simulink model "limit_detection_test"  (R2013a)
settings: Solver=ode3  StartTime=0  StopTime=10000  FixedStep=1  RelTol=1e-3
libraries: simulink x1
settings Model: Creator=sfrank1  LastModifiedBy=sfrank1

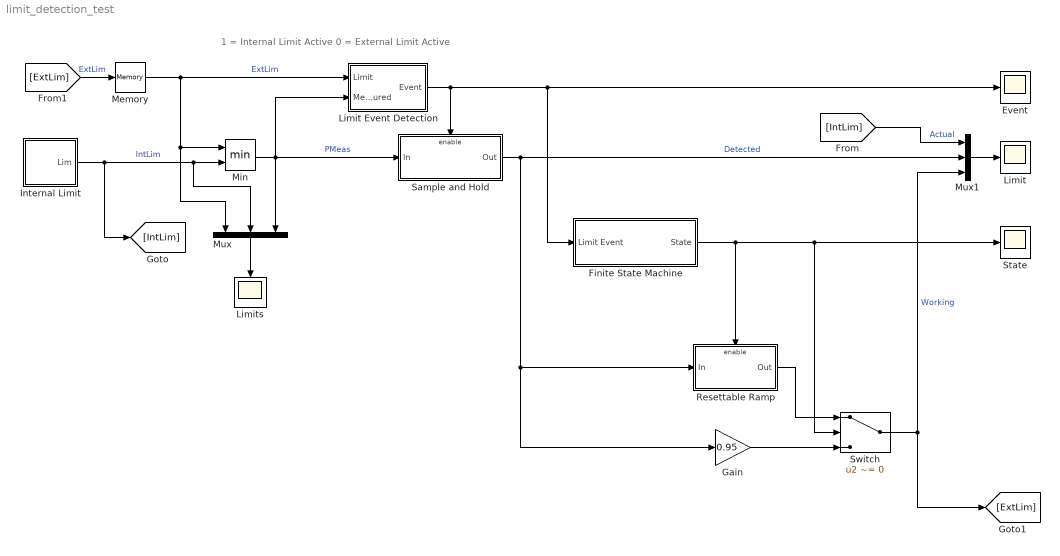
== system limit_detection_test ==
  note: 1 = Internal Limit Active
      | 0 = External Limit Active
  Event : Scope
      settings: TimeRange=10000  YMin=0  YMax=1
  Finite State Machine : Subsystem  TreatAsAtomicUnit=on
      settings: RTWFcnNameOpts=Use subsystem name  RTWFileNameOpts=Use function name
  Gain : Gain  Gain=0.95
  Internal Limit : Subsystem  TreatAsAtomicUnit=on
      settings: RTWFcnNameOpts=Use subsystem name  RTWFileNameOpts=Use function name
  Limit : Scope
      settings: ShowLegends=on  TimeRange=10000  YMin=0  YMax=2000  SaveName=ScopeData2
  Limit Event Detection : Subsystem  TreatAsAtomicUnit=on
      settings: RTWFcnNameOpts=Use subsystem name  RTWFileNameOpts=Use function name
  Limits : Scope
      settings: ShowLegends=on  TimeRange=10000  YMin=0  YMax=2000
  Memory : Memory
  Min : MinMax  Inputs=2
  Mux : Mux  Inputs=3
  Mux1 : Mux  Inputs=3
  Resettable Ramp : Subsystem  TreatAsAtomicUnit=on
  Sample and Hold : Subsystem  TreatAsAtomicUnit=on
  State : Scope
      settings: TimeRange=10000  YMin=0  YMax=1  SaveName=ScopeData4
  Switch : Switch  Criteria=u2 ~= 0
  wires:
  [ExtLim] -> Memory/1  "ExtLim"
  Min/1 -> Mux/3, Sample and Hold/1(In), Limit Event Detection/2(Measured)  "PMeas"
  Limit Event Detection/1(Event) -> Finite State Machine/1(Limit Event), Event/1, Sample and Hold/Enable
  Internal Limit/1(Lim) -> [IntLim], Mux/2, Min/2  "IntLim"
  Mux/1 -> Limits/1
  Finite State Machine/1(State) -> Switch/2, State/1, Resettable Ramp/Enable
  Resettable Ramp/1(Out) -> Switch/1
  Switch/1 -> [ExtLim], Mux1/3  "Working"
  Mux1/1 -> Limit/1
  [IntLim] -> Mux1/1  "Actual"
  Sample and Hold/1(Out) -> Mux1/2, Resettable Ramp/1(In), Gain/1  "Detected"
  Memory/1 -> Limit Event Detection/1(Limit), Mux/1, Min/1  "ExtLim"
  Gain/1 -> Switch/3

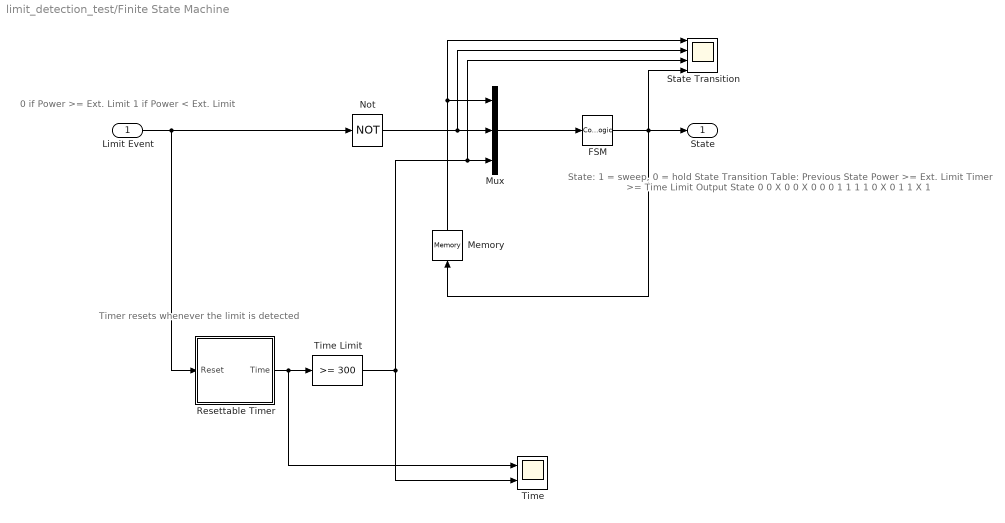
== system limit_detection_test/Finite State Machine ==
  note: Timer resets whenever the limit is detected
  note: 0 if Power >= Ext. Limit
      | 1 if Power < Ext. Limit
  note: State: 1 = sweep, 0 = hold
      |
      | State Transition Table:
      |
      | Previous State	Power >= Ext. Limit	Timer  >= Time Limit		Output State
      | 0				0					X						0
      | 0				X					0						0
      | 0				1					1						1
      | 1				0					X						0
      | 1				1					X						1
  Limit Event : Inport
  FSM : CombinatorialLogic  TruthTable=[0; 0; 0; 1; 0; 0; 1; 1]
  Memory : Memory  X0=1
  Mux : Mux  Inputs=3
  Not : Logic  Operator=NOT  IconShape=distinctive  AllPortsSameDT=off  OutDataTypeStr=boolean
  Resettable Timer : Subsystem  TreatAsAtomicUnit=on
  State Transition : Scope  NumInputPorts=4
      settings: TimeRange=10000  YMin=0~0~0~0  YMax=1~1~1~1  SaveName=ScopeData6
  Time : Scope  NumInputPorts=2
      settings: TimeRange=10000  YMin=0~-5  YMax=3500~5  SaveName=ScopeData5
  Time Limit : simulink/Logic and Bit Operations/Compare To Constant  relop=>=  const=300  OutDataTypeStr=boolean
  State : Outport
  wires:
  FSM/1 -> Memory/1, State/1, State Transition/4
  Limit Event/1 -> Resettable Timer/1(Reset), Not/1
  Not/1 -> State Transition/2, Mux/2
  Mux/1 -> FSM/1
  Time Limit/1 -> Time/2, State Transition/3, Mux/3
  Memory/1 -> State Transition/1, Mux/1
  Resettable Timer/1(Time) -> Time/1, Time Limit/1

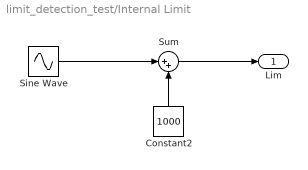
== system limit_detection_test/Internal Limit ==
  Constant2 : Constant  Value=1000
  Sine Wave : Sin  Amplitude=500  Frequency=1/900  SampleTime=0
  Sum : Sum  Inputs=|++
  Lim : Outport
  wires:
  Constant2/1 -> Sum/2
  Sum/1 -> Lim/1
  Sine Wave/1 -> Sum/1

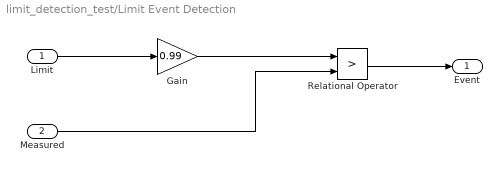
== system limit_detection_test/Limit Event Detection ==
  Limit : Inport
  Measured : Inport  Port=2
  Gain : Gain  Gain=0.99
  Relational Operator : RelationalOperator  Operator=>  OutDataTypeStr=boolean
  Event : Outport
  wires:
  Gain/1 -> Relational Operator/1
  Limit/1 -> Gain/1
  Relational Operator/1 -> Event/1
  Measured/1 -> Relational Operator/2

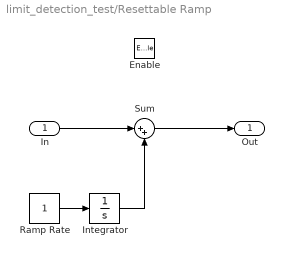
== system limit_detection_test/Resettable Ramp ==
  In : Inport
  Enable : EnablePort  StatesWhenEnabling=reset
  Integrator : Integrator
  Ramp Rate : Constant
  Sum : Sum  Inputs=|++
  Out : Outport
  wires:
  In/1 -> Sum/1
  Sum/1 -> Out/1
  Ramp Rate/1 -> Integrator/1
  Integrator/1 -> Sum/2

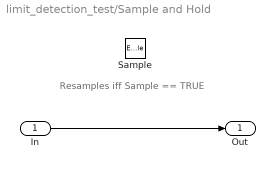
== system limit_detection_test/Sample and Hold ==
  note: Resamples iff Sample == TRUE
  In : Inport
  Sample : EnablePort
  Out : Outport
  wires:
  In/1 -> Out/1

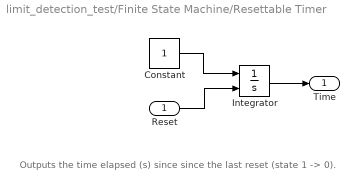
== system limit_detection_test/Finite State Machine/Resettable Timer ==
  note: Outputs the time elapsed (s) since
      | since the last reset (state 1 -> 0).
  Reset : Inport
  Constant : Constant
  Integrator : Integrator  ExternalReset=level
  Time : Outport
  wires:
  Constant/1 -> Integrator/1
  Integrator/1 -> Time/1
  Reset/1 -> Integrator/2
